simulink model "dc_motor_sim"  (R2016b)
settings: Solver=VariableStepAuto  StartTime=0.0  StopTime=10  RelTol=1e-3
libraries: powerlib x3
settings Model: Creator=USER  LastModifiedBy=USER
settings DebuggingCC: MaxConsecutiveZCsMsg=none

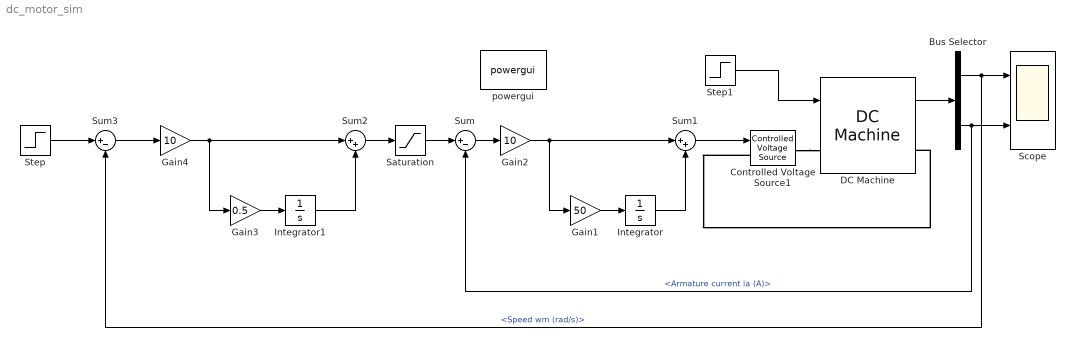
== system dc_motor_sim ==
  Bus Selector : BusSelector  OutputSignals=Speed wm (rad/s),Armature current ia (A)
  Controlled Voltage Source1 : powerlib/Electrical Sources/Controlled Voltage Source  Initialize=on  Source_Type=AC  Amplitude=0  Phase=0  Frequency=0  Measurements=None
  DC Machine : powerlib/Machines/DC Machine  PresetModel=No  MechanicalLoad=Speed w  FieldType=Permanent magnet  ShowDetailedParameters=on  MeasurementBus=off  RLa="[ 0.6  0.012]"  RLf="[ 240  120]"  Laf=1.8  MachineConstant=Torque constant (N.m/A)  Ke=1.8  Kt=1.8  J=1  Bm=0.1  Tf=0  w0=0  Ifinit=1  TsPowergui=0  TsBlock=-1
  Gain1 : Gain  Gain=50
  Gain2 : Gain  Gain=10
  Gain3 : Gain  Gain=0.5
  Gain4 : Gain  Gain=10
  Integrator : Integrator
  Integrator1 : Integrator
  Saturation : Saturate  UpperLimit=4  LowerLimit=-4
  Scope : Scope  NumInputPorts=2
  Step : Step  Time=0.2  After=2  SampleTime=0
  Step1 : Step  Time=5  After=0  SampleTime=0
  Sum : Sum  Inputs=|+-
  Sum1 : Sum  Inputs=|++
  Sum2 : Sum  Inputs=|++
  Sum3 : Sum  Inputs=|+-
  powergui : powerlib/powergui  Priority=1  SimulationMode=Continuous  SolverType=Tustin/Backward Euler (TBE)  SampleTime=50e-6  frequency=60  SPID=off  DisableSnubberDevices=off  DisableRonSwitches=off  DisableVfSwitches=off  SwTol=0  DisplayEquations=off  Interpol=off  ExternalGateDelay=off  methode=off  Ts=10  FunctionMessages=off  echomessages=off  HookPort=off  EnableUseOfTLC=off  x0status=blocks  frequencyindice=0  Pbase=100e6  ErrMax=1e-4  Iterations=50  UnitsV=kV  UnitsW=MW  buscounter=0  RestoreLinks=warning  ResistiveCurrentMeasurement=off  Frange=[0:2:500]  Ylog=off  Xlog=on  ShowGrid=off  save=off  variable=ZData  structure=0  ZoomFFT=off  StartTime=0.0  cycles=1  DisplayStyle=1  fundamental=60  FreqAxis=off  MaxFrequency=1000  frequencyindicesteady=1  RmsSteady=1  display=off
  wires:
  DC Machine/1 -> Bus Selector/1
  Sum1/1 -> Controlled Voltage Source1/1
  Sum/1 -> Gain2/1
  Gain1/1 -> Integrator/1
  Integrator/1 -> Sum1/2
  Gain2/1 -> Sum1/1, Gain1/1
  Step1/1 -> DC Machine/1
  Bus Selector/2 -> Scope/2, Sum/2  "<Armature current ia (A)>"
  Sum2/1 -> Saturation/1
  Sum3/1 -> Gain4/1
  Gain3/1 -> Integrator1/1
  Gain4/1 -> Sum2/1, Gain3/1
  Integrator1/1 -> Sum2/2
  Bus Selector/1 -> Scope/1, Sum3/2  "<Speed wm (rad/s)>"
  Step/1 -> Sum3/1
  Saturation/1 -> Sum/1
  connections:
  Controlled Voltage Source1/RConn1 -- DC Machine/LConn1
  Controlled Voltage Source1/LConn1 -- DC Machine/RConn1
